simulink model "motorAndEncoderTest"  (R2015a)
settings: Solver=ode3  StartTime=0.0  StopTime=5  RelTol=1e-3
settings Model: SimulationMode=external  ExtModeTrigDuration=100  Creator=Justin  LastModifiedBy=Justin
settings OptimizationCC: OptimizeModelRefInitCode=on  LifeSpan=Inf
settings HardwareCC: ProdLargestAtomicInteger=Long  ProdLargestAtomicFloat=Double  ProdEndianess=LittleEndian  ProdHWDeviceType=ARM Compatible->ARM Cortex
settings RTWCC: SystemTargetFile=realtime.tlc  GenerateMakefile=off  TemplateMakefile=realtime.tmf  Description=Run on Target Hardware  RTWVerbose=off
settings ERTTargetCC: CombineOutputUpdateFcns=off  ERTSrcFileBannerTemplate=realtime_code_template.cgt  ERTHdrFileBannerTemplate=realtime_code_template.cgt  ERTDataSrcFileTemplate=realtime_code_template.cgt  ERTDataHdrFileTemplate=realtime_code_template.cgt  ERTCustomFileTemplate=realtime_file_process.tlc

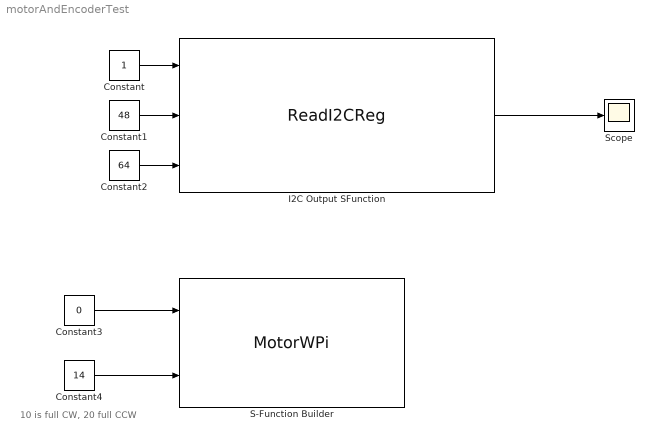
== system motorAndEncoderTest ==
  note: 10 is full CW, 20 full CCW
  Constant : Constant  OutDataTypeStr=uint8
  Constant1 : Constant  Value=48  OutDataTypeStr=uint8
  Constant2 : Constant  Value=64  OutDataTypeStr=uint8
  Constant3 : Constant  Value=0  OutDataTypeStr=uint8
  Constant4 : Constant  Value=14  OutDataTypeStr=uint8
  I2C Output SFunction : S-Function  InitFcn=try, set_param(gcb,'FunctionName','ReadI2CReg'), end  FunctionName=ReadI2CReg  SFunctionModules=ReadI2CReg_wrapper  mask(S-Function Builder){}
      mask init:
      | val = [[.9  0.75 0.75 1 1 .9 .9 1]',[1 1 0.75 0.75 .9 .9 1 .9]'];try , sys = get_param(gcb,'SfunBuilderFcnName');if isempty(sys), sys = get_param(gcb,'FunctionName'); end,catch, sys = get_param(gcb,'FunctionName'); end
      settings: CopyFcn=set_param(gcbh,'LinkStatus','none')  PreSaveFcn=try, set_param(gcb,'FunctionName','ReadI2CReg'), end  OpenFcn=sfunctionwizard(gcbh)
      mask Display:
      | plot(val(:,1),val(:,2))
      | disp(sys)
      | port_label('input',1,'Bus_Number')
      | port_label('input',2,'Device_Address')
      | port_label('input',3,'Register_Address')
      | port_label('output',1,'Register_Value')
  S-Function Builder : S-Function  InitFcn=try, set_param(gcb,'FunctionName','MotorWPi'), end  FunctionName=MotorWPi  SFunctionModules=MotorWPi_wrapper  mask(S-Function Builder){}
      mask help: Simulink:masks:SFunctionBuilder_MD
      mask init: same as motorAndEncoderTest/I2C Output SFunction
      settings: CopyFcn=set_param(gcbh,'LinkStatus','none')  PreSaveFcn=try, set_param(gcb,'FunctionName','MotorWPi'), end  OpenFcn=sfunctionwizard(gcbh)
      mask Display: plot(val(:,1),val(:,2)),disp(sys), port_label('input',1,'GPIO_Number'), port_label('input',2,'GPIO_Value')
  Scope : Scope
      settings: YMin=0  YMax=4.5e+09
  wires:
  I2C Output SFunction/1 -> Scope/1
  Constant/1 -> I2C Output SFunction/1
  Constant2/1 -> I2C Output SFunction/3
  Constant1/1 -> I2C Output SFunction/2
  Constant3/1 -> S-Function Builder/1
  Constant4/1 -> S-Function Builder/2
